simulink library "vmc"  (R2021b)
settings: Solver=VariableStepAuto  StartTime=0.0  StopTime=10.0  RelTol=1e-3
undefined symbols (not defined in the file or in its folder): AVMC_ACCDeltaTqIGain_X_kph, AVMC_ACCDeltaTqIGain_Y_mps2, AVMC_ACCDeltaTqPGain_X_kph, AVMC_ACCDeltaTqPGain_Y_kph, AVMC_ACCLongSteadyCtrl_X_kph, AVMC_AggressJerkPCT4AT_X_kph, AVMC_AggressJerkPCT_X_kph, AVMC_AggressLimitPCT4AT_X_kph, AVMC_AggressLimitPCT_X_kph, AVMC_CCLongSteadyCtrl_X_kph, AVMC_DISCDeltaTqIGain_X_kph, AVMC_DISCDeltaTqIGain_Y_mps2, AVMC_DISCDeltaTqPGain_X_kph, AVMC_DISCDeltaTqPGain_Y_kph, AVMC_DISCTrunAccJerk_X_s, AVMC_DISCTrunAccLimit_X_s, AVMC_ESCRegenOut_X_kph, AVMC_ESCRegenOut_Y_Deg, AVMC_ESCRegenOutEnSpd_X_Deg, AVMC_ISOAccLimit_X_mps, AVMC_ISODecLimit_X_mps, AVMC_ISOJerk_X_mps, AVMC_LatESCRegenOut_X_kph, AVMC_LatESCRegenOut_Y_Deg, AVMC_LongAccDeadZone_X_kph, AVMC_LongAccFiltTsforP2_X_Gps, AVMC_MCPresBaseTq_X_bar, AVMC_MSALongSteadyCtrl_X_kph, AVMC_MSAPedalOvrd2_X_kph, AVMC_MSAPedalOvrd_X_kph, AVMC_MSASpdBand_X_kph, AVMC_MSATqDownEndTq_X_kph, AVMC_MSATqDownTime_X_kph, AVMC_RDCDetectTime_X_kph, AVMC_RDCDetectTime_Y_pct, AVMC_RDCEnSlideRate_X_Deg, AVMC_RearWhlTqRatio_X_Nm, AVMC_RearWhlTqRatio_Y_gps, AVMC_RearWhlTqSlipGain_X_rat, AVMC_RearWhlTqSlipGain_Y_kph, AVMC_SoftJerkPCT_X_kph, AVMC_SoftLimitPCT_X_kph, AVMC_StESCYaw_X_kph, AVMC_StESCYaw_Y_Deg, AVMC_StESCYawCom_X_kph, AVMC_StESCYawCom_Y_Gps, AVMC_TMSpdBaseTq_X_rpm, AVMC_VehHoldBDecMap_X_kph, AVMC_VehHoldDecCtrlTime_X_kph, AVMC_VehHoldMCPPass_X_deg, C_TASK_10MS_S, C_TASK_5MS_S, DEG2RAD, Discrete, ENUM_ACCAVAIL_AVAILABLE, ENUM_ACCCTRLALLOW_ALLOW, ENUM_ADASACCSTA_ACTIVE, ENUM_ADASACCSTA_OVERRIDE, ENUM_ADASACCSTA_SHUTOFF, ENUM_ADASAEBREQ_NOREQUEST ... (+361)
libraries: hcu_lib x63, simulink x60, simulink_extras x3, ctrlSharedLib x3, $bdroot x2
(part 15 of 15)

== stateflow chart vmc/VMC/VMC/SafetyControl/SafetyControlJudgement/SingleWheelSlipRatio/SingleWheelSlipRatioJudgement ==
  state SingleWheelSlipRatioJudgement
    (default) -> (junction 14) : {VVMC_SingleWhlSlipRatioCtrl_flg = FALSE}
    SingleWheelSlipRatioJudgement -> (junction 14)
    (junction 14) -> (junction 105) [order 1] : [VINP_LFRawWhlSpeedV_flg == FALSE]
    (junction 105) -> (junction 117) [order 1] : [abs(VINP_VehSpeed_kph - VVMC_LFWhlSpeedRollAve_kph) >= KVMC_SingleWhlSlipRatioTHR_kph]
    (junction 14) -> (junction 121) [order 2]
    (junction 105) -> (junction 119) [order 2]
    (junction 117) -> (junction 107) : {VVMC_SingleWhlSlipRatioCtrl_flg = TRUE}
    (junction 119) -> (junction 121)
    (junction 121) -> (junction 134)
    (junction 134) -> (junction 130) [order 1] : [VINP_RFRawWhlSpeedV_flg == FALSE]
    (junction 130) -> (junction 125) [order 1] : [abs(VINP_VehSpeed_kph - VVMC_RFWhlSpeedRollAve_kph) >= KVMC_SingleWhlSlipRatioTHR_kph]
    (junction 134) -> (junction 127) [order 2]
    (junction 130) -> (junction 132) [order 2]
    (junction 125) -> (junction 131) : {VVMC_SingleWhlSlipRatioCtrl_flg = TRUE}
    (junction 132) -> (junction 127)
    (junction 127) -> (junction 143)
    (junction 143) -> (junction 149) [order 1] : [VINP_LRRawWhlSpeedV_flg == FALSE]
    (junction 149) -> (junction 144) [order 1] : [abs(VINP_VehSpeed_kph - VVMC_LRWhlSpeedRollAve_kph) >= KVMC_SingleWhlSlipRatioTHR_kph]
    (junction 143) -> (junction 137) [order 2]
    (junction 149) -> (junction 146) [order 2]
    (junction 144) -> (junction 148) : {VVMC_SingleWhlSlipRatioCtrl_flg = TRUE}
    (junction 146) -> (junction 137)
    (junction 137) -> (junction 154)
    (junction 154) -> (junction 153) [order 1] : [VINP_RRRawWhlSpeedV_flg == FALSE]
    (junction 153) -> (junction 150) [order 1] : [abs(VINP_VehSpeed_kph - VVMC_RRWhlSpeedRollAve_kph) >= KVMC_SingleWhlSlipRatioTHR_kph]
    (junction 154) -> (junction 169) [order 2]
    (junction 153) -> (junction 152) [order 2]
    (junction 150) -> (junction 155) : {VVMC_SingleWhlSlipRatioCtrl_flg = TRUE}
    (junction 152) -> (junction 169)
    (junction 169) -> (junction 157)
    (junction 157) -> (junction 163) [order 1] : [(VINP_LFRawWhlSpeedV_flg == TRUE &&...
        |   VINP_RFRawWhlSpeedV_flg == TRUE) ||...
        |  (VINP_LRRawWhlSpeedV_flg == TRUE &&...
        |   VINP_RRRawWhlSpeedV_flg == TRUE)]
    (junction 157) -> (junction 167) [order 2] : {VVMC_SingleWhlSlipRatioCtrl_flg = FALSE}
    (junction 163) -> (junction 165) : {VVMC_SingleWhlSlipRatioCtrl_flg = TRUE}
  data: VINP_VehSpeed_kph input single; VVMC_LFWhlSpeedRollAve_kph input single; VVMC_RFWhlSpeedRollAve_kph input single; VVMC_LRWhlSpeedRollAve_kph input single; VVMC_RRWhlSpeedRollAve_kph input single; VINP_LFRawWhlSpeedV_flg input boolean; VINP_RFRawWhlSpeedV_flg input boolean; VINP_LRRawWhlSpeedV_flg input boolean; VINP_RRRawWhlSpeedV_flg input boolean; KVMC_SingleWhlSlipRatioTHR_kph input single; TRUE input boolean; VVMC_SingleWhlSlipRatioCtrl_flg output boolean; FALSE input boolean

== stateflow chart vmc/VMC/VMC/SpeedArbitration/Response Gain/Response Gain ==
  state ResponseGain
    (default) -> (junction 81) : {VVMC_JerkPCT_pct = ZERO_FLOAT;
        |  VVMC_LimitPCT_pct = ZERO_FLOAT}
    ResponseGain -> (junction 81)
    (junction 81) -> (junction 73) [order 1] : [VVMC_FeatArbitrSta_enum == ENUM_FEATARBITRSTA_DISC ||...
        |  VVMC_FeatArbitrSta_enum == ENUM_FEATARBITRSTA_CC ||...
        |  VVMC_FeatArbitrSta_enum == ENUM_FEATARBITRSTA_MSA ||...
        |  VVMC_FeatArbitrSta_enum == ENUM_FEATARBITRSTA_ACCDISC]
    (junction 73) -> (junction 75) [order 1] : [VDSC_DISCTurn_flg == ENUM_DISCTURN_ACTIVE ||...
        | (VVMC_FeatArbitrSta_enum == ENUM_FEATARBITRSTA_MSA &&...
        |  KVMC_MSAResponseAGSV_flg == TRUE)]
    (junction 81) -> (junction 92) [order 2] : {VVMC_JerkPCT_pct = ZERO_FLOAT;
        |  VVMC_LimitPCT_pct = ZERO_FLOAT}
    (junction 73) -> (junction 77) [order 2] : {VVMC_JerkPCT_pct = VVMC_SoftJerkPCT_pct;
        |  VVMC_LimitPCT_pct = VVMC_SoftLimitPCT_pct}
    (junction 75) -> (junction 78) : {VVMC_JerkPCT_pct = VVMC_AggressJerkPCT_pct;
        |  VVMC_LimitPCT_pct = VVMC_AggressLimitPCT_pct}
  data: VDSC_DISCTurn_flg input uint8; VVMC_FeatArbitrSta_enum input uint8; VVMC_JerkPCT_pct output single; VVMC_LimitPCT_pct output single; VVMC_SoftJerkPCT_pct input single; VVMC_AggressJerkPCT_pct input single; VVMC_SoftLimitPCT_pct input single; VVMC_AggressLimitPCT_pct input single; ENUM_FEATARBITRSTA_DISC input uint8; ENUM_FEATARBITRSTA_CC input; ZERO_FLOAT input single; ENUM_DISCTURN_ACTIVE input uint8; ENUM_FEATARBITRSTA_ACCDISC input uint8; ENUM_FEATARBITRSTA_MSA input; TRUE input; KVMC_MSAResponseAGSV_flg input

== stateflow chart vmc/VMC/VMC/SpeedArbitration/Feature Status Confirm/Feature Status Confirm ==
  state FeatStaConfrim
    (default) -> (junction 197) : {VVMC_FeatStaConfirm_enum = ENUM_FEATSTACFM_INACTIVE}
    FeatStaConfrim -> (junction 197)
    (junction 197) -> (junction 203) [order 1] : [VVMC_VMCAEBCtrlAvail_flg == ENUM_VMCAEBCTRLAVAIL_AVAILABLE &&...
        | (VINP_ADASAEBSta_enum == ENUM_ADASAEBSTA_ACTIVE ||...
        |  VINP_ADASAEBReq_enum ~= ENUM_ADASAEBREQ_NOREQUEST)]
    (junction 197) -> (junction 200) [order 2]
    (junction 203) -> (junction 202) : {VVMC_FeatStaConfirm_enum = ENUM_FEATSTACFM_AEB}
    (junction 200) -> (junction 208) [order 1] : [VVMC_VMCACCCtrlAvail_flg == ENUM_VMCACCCTRLAVAIL_AVAILABLE &&...
        |  VDSC_DISCSta_enum == ENUM_DISCSTA_ACTIVE]
    (junction 208) -> (junction 210) [order 1] : [VINP_ADASACCSta_enum == ENUM_ADASACCSTA_ACTIVE ||...
        |  VINP_ADASACCSta_enum == ENUM_ADASACCSTA_SHUTOFF ||...
        |  VINP_ADASACCSta_enum == ENUM_ADASACCSTA_OVERRIDE]
    (junction 200) -> (junction 232) [order 2]
    (junction 208) -> (junction 214) [order 2]
    (junction 210) -> (junction 212) : {VVMC_FeatStaConfirm_enum = ENUM_FEATSTACFM_ACCDISC}
    (junction 214) -> (junction 216) [order 1] : [(VVMC_CCCtrlSta_enum == ENUM_CCCRLSTA_ACTIVE ||...
        |   VVMC_CCCtrlSta_enum == ENUM_CCCRLSTA_OVERRIDE) &&...
        |  VVMC_VMCCCCtrlAvail_flg == ENUM_VMCCCCTRLAVAIL_AVAILABLE]
    (junction 214) -> (junction 222) [order 2]
    (junction 216) -> (junction 218) : {VVMC_FeatStaConfirm_enum = ENUM_FEATSTACFM_CCDISC}
    (junction 222) -> (junction 224) [order 1] : [(VVMC_MSACtrlSta_enum == ENUM_MSACRLSTA_ACTIVE ||...
        |   VVMC_MSACtrlSta_enum == ENUM_MSACRLSTA_OVERRIDE) &&...
        |  VVMC_VMCMSACtrlAvail_flg == ENUM_VMCMSACTRLAVAIL_AVAILABLE]
    (junction 222) -> (junction 229) [order 2] : {VVMC_FeatStaConfirm_enum = ENUM_FEATSTACFM_DISC}
    (junction 224) -> (junction 221) : {VVMC_FeatStaConfirm_enum = ENUM_FEATSTACFM_DISCMSA}
    (junction 232) -> (junction 234) [order 1] : [VVMC_VMCACCCtrlAvail_flg == ENUM_VMCACCCTRLAVAIL_AVAILABLE &&...
        | (VINP_ADASACCSta_enum == ENUM_ADASACCSTA_ACTIVE ||...
        |  VINP_ADASACCSta_enum == ENUM_ADASACCSTA_OVERRIDE ||...
        |  VINP_ADASACCSta_enum == ENUM_ADASACCSTA_SHUTOFF)]
    (junction 232) -> (junction 238) [order 2]
    (junction 234) -> (junction 236) : {VVMC_FeatStaConfirm_enum = ENUM_FEATSTACFM_ACC}
    (junction 238) -> (junction 240) [order 1] : [(VVMC_CCCtrlSta_enum == ENUM_CCCRLSTA_ACTIVE ||...
        |   VVMC_CCCtrlSta_enum == ENUM_CCCRLSTA_OVERRIDE) &&...
        |  VVMC_VMCCCCtrlAvail_flg == ENUM_VMCCCCTRLAVAIL_AVAILABLE]
    (junction 238) -> (junction 250) [order 2]
    (junction 240) -> (junction 244) : {VVMC_FeatStaConfirm_enum = ENUM_FEATSTACFM_CC}
    (junction 250) -> (junction 249) [order 1] : [(VVMC_MSACtrlSta_enum == ENUM_MSACRLSTA_ACTIVE ||...
        |   VVMC_MSACtrlSta_enum == ENUM_MSACRLSTA_OVERRIDE) &&...
        |  VVMC_VMCMSACtrlAvail_flg == ENUM_VMCMSACTRLAVAIL_AVAILABLE]
    (junction 250) -> (junction 252) [order 2] : {VVMC_FeatStaConfirm_enum = ENUM_FEATSTACFM_INACTIVE}
    (junction 249) -> (junction 248) : {VVMC_FeatStaConfirm_enum = ENUM_FEATSTACFM_MSA}
  data: VVMC_VMCCCCtrlAvail_flg input boolean; ENUM_VMCCCCTRLAVAIL_AVAILABLE input uint8; VVMC_VMCMSACtrlAvail_flg input boolean; ENUM_VMCMSACTRLAVAIL_AVAILABLE input uint8; VVMC_VMCAEBCtrlAvail_flg input boolean; ENUM_VMCAEBCTRLAVAIL_AVAILABLE input uint8; VVMC_VMCACCCtrlAvail_flg input boolean; ENUM_VMCACCCTRLAVAIL_AVAILABLE input uint8; VINP_ADASAEBSta_enum input uint8; VDSC_DISCSta_enum input uint8; VINP_ADASACCSta_enum input uint8; VVMC_CCCtrlSta_enum input uint8; VVMC_FeatStaConfirm_enum output uint8; VVMC_MSACtrlSta_enum input uint8; ENUM_FEATSTACFM_INACTIVE input uint8; ENUM_FEATSTACFM_AEB input uint8; ENUM_FEATSTACFM_ACC input uint8; ENUM_FEATSTACFM_CC input uint8; ENUM_FEATSTACFM_DISC input uint8; ENUM_FEATSTACFM_MSA input uint8; ENUM_FEATSTACFM_ACCDISC input uint8; ENUM_FEATSTACFM_CCDISC input uint8; ENUM_FEATSTACFM_DISCMSA input uint8; ENUM_ADASAEBSTA_ACTIVE input uint8; ENUM_ADASACCSTA_ACTIVE input uint8; ENUM_ADASACCSTA_SHUTOFF input uint8; ENUM_CCCRLSTA_ACTIVE input uint8; ENUM_MSACRLSTA_ACTIVE input uint8; ENUM_DISCSTA_ACTIVE input uint8; ENUM_ADASACCSTA_OVERRIDE input uint8; VINP_ADASAEBReq_enum input uint8; ENUM_ADASAEBREQ_NOREQUEST input uint8; ENUM_CCCRLSTA_OVERRIDE input; ENUM_MSACRLSTA_OVERRIDE input

== stateflow chart vmc/VMC/VMC/SpeedArbitration/Feature Arbitration/Feature Arbitration ==
  state FeatureArbitration
    (default) -> (junction 406) : {VVMC_FeatArbitrSta_enum = ENUM_FEATARBITRSTA_INACTIVE;
        |  VVMC_FeatReqSpd_kph = ZERO_FLOAT;}
    FeatureArbitration -> (junction 406)
    (junction 406) -> (junction 409) [order 1] : [VVMC_FeatStaConfirm_enum == ENUM_FEATSTACFM_AEB]
    (junction 406) -> (junction 413) [order 2]
    (junction 409) -> (junction 411) : {VVMC_FeatArbitrSta_enum = ENUM_FEATARBITRSTA_AEB;
        |  VVMC_FeatReqSpd_kph = ZERO_FLOAT}
    (junction 413) -> (junction 415) [order 1] : [VVMC_FeatStaConfirm_enum == ENUM_FEATSTACFM_ACC]
    (junction 413) -> (junction 430) [order 2]
    (junction 415) -> (junction 417) : {VVMC_FeatArbitrSta_enum = ENUM_FEATARBITRSTA_ACC;
        |  VVMC_FeatReqSpd_kph = ZERO_FLOAT}
    (junction 430) -> (junction 431) [order 1] : [VVMC_FeatStaConfirm_enum == ENUM_FEATSTACFM_CC]
    (junction 430) -> (junction 440) [order 2]
    (junction 431) -> (junction 433) : {VVMC_FeatArbitrSta_enum = ENUM_FEATARBITRSTA_CC;
        |  VVMC_FeatReqSpd_kph = VVMC_FeatSetSpdForCalcu_kph}
    (junction 440) -> (junction 441) [order 1] : [VVMC_FeatStaConfirm_enum == ENUM_FEATSTACFM_DISC]
    (junction 440) -> (junction 445) [order 2]
    (junction 441) -> (junction 438) : {VVMC_FeatArbitrSta_enum = ENUM_FEATARBITRSTA_DISC;
        |  VVMC_FeatReqSpd_kph = VDSC_DISCTargetSpd_kph}
    (junction 445) -> (junction 443) [order 1] : [VVMC_FeatStaConfirm_enum == ENUM_FEATSTACFM_MSA]
    (junction 445) -> (junction 449) [order 2]
    (junction 443) -> (junction 444) : {VVMC_FeatArbitrSta_enum = ENUM_FEATARBITRSTA_MSA;
        |  VVMC_FeatReqSpd_kph = VVMC_FeatSetSpdForCalcu_kph}
    (junction 449) -> (junction 450) [order 1] : [VVMC_FeatStaConfirm_enum == ENUM_FEATSTACFM_ACCDISC]
    (junction 450) -> (junction 557) [order 1] : [VVMC_FeatSetSpdForCalcu_kph <= VDSC_DISCTargetSpd_kph]
    (junction 557) -> (junction 551) [order 1] : [VVMC_FeatSetSpdForCalcu_kph < VDSC_DISCTargetSpd_kph]
    (junction 449) -> (junction 512) [order 2]
    (junction 450) -> (junction 467) [order 2] : {VVMC_FeatArbitrSta_enum = ENUM_FEATARBITRSTA_ACCDISC;
        |  VVMC_FeatReqSpd_kph = VDSC_DISCTargetSpd_kph}
    (junction 557) -> (junction 559) [order 2]
    (junction 551) -> (junction 553) : {VVMC_FeatArbitrSta_enum = ENUM_FEATARBITRSTA_ACC;
        |  VVMC_FeatReqSpd_kph = ZERO_FLOAT}
    (junction 559) -> (junction 561) [order 1] : [VVMC_LastFeatArbitrFinal_enum != ENUM_FEATARBITRSTA_DISC]
    (junction 559) -> (junction 565) [order 2]
    (junction 561) -> (junction 564) : {VVMC_FeatArbitrSta_enum = ENUM_FEATARBITRSTA_ACC;
        |  VVMC_FeatReqSpd_kph = ZERO_FLOAT}
    (junction 565) -> (junction 567) [order 1] : [VVMC_LastActACCRequiredAccel_mps2 > ZERO_FLOAT ||...
        |  VVMC_LastActACCRequiredAccel_mps2 < ZERO_FLOAT ]
    (junction 565) -> (junction 569) [order 2] : {VVMC_FeatArbitrSta_enum = ENUM_FEATARBITRSTA_ACC;
        |  VVMC_FeatReqSpd_kph = ZERO_FLOAT}
    (junction 567) -> (junction 572) : {VVMC_FeatArbitrSta_enum = ENUM_FEATARBITRSTA_DISC;
        |  VVMC_FeatReqSpd_kph = VDSC_DISCTargetSpd_kph}
    (junction 512) -> (junction 514) [order 1] : [VVMC_FeatStaConfirm_enum == ENUM_FEATSTACFM_CCDISC ||...
        |  VVMC_FeatStaConfirm_enum == ENUM_FEATSTACFM_DISCMSA]
    (junction 514) -> (junction 516) [order 1] : [VVMC_FeatSetSpdForCalcu_kph < VDSC_DISCTargetSpd_kph]
    (junction 516) -> (junction 518) [order 1] : [VVMC_FeatStaConfirm_enum == ENUM_FEATSTACFM_CCDISC]
    (junction 512) -> (junction 527) [order 2] : {VVMC_FeatArbitrSta_enum = ENUM_FEATARBITRSTA_INACTIVE;
        |  VVMC_FeatReqSpd_kph = ZERO_FLOAT}
    (junction 514) -> (junction 525) [order 2] : {VVMC_FeatArbitrSta_enum = ENUM_FEATARBITRSTA_DISC;
        |  VVMC_FeatReqSpd_kph = VDSC_DISCTargetSpd_kph}
    (junction 516) -> (junction 522) [order 2] : {VVMC_FeatArbitrSta_enum = ENUM_FEATARBITRSTA_MSA;
        |  VVMC_FeatReqSpd_kph = VVMC_FeatSetSpdForCalcu_kph}
    (junction 518) -> (junction 520) : {VVMC_FeatArbitrSta_enum = ENUM_FEATARBITRSTA_CC;
        |  VVMC_FeatReqSpd_kph = VVMC_FeatSetSpdForCalcu_kph}
  data: VVMC_FeatStaConfirm_enum input uint8; VDSC_DISCTargetSpd_kph input single; VVMC_FeatSetSpdForCalcu_kph input single; VVMC_FeatArbitrSta_enum output uint8; VVMC_FeatReqSpd_kph output single; ENUM_FEATSTACFM_AEB input uint8; ENUM_FEATSTACFM_ACC input uint8; ENUM_FEATSTACFM_CC input uint8; ENUM_FEATSTACFM_DISC input uint8; ENUM_FEATSTACFM_MSA input uint8; ENUM_FEATSTACFM_ACCDISC input uint8; ENUM_FEATSTACFM_CCDISC input uint8; ENUM_FEATSTACFM_DISCMSA input uint8; ENUM_FEATARBITRSTA_INACTIVE input uint8; ENUM_FEATARBITRSTA_AEB input uint8; ENUM_FEATARBITRSTA_ACC input uint8; ENUM_FEATARBITRSTA_CC input uint8; ENUM_FEATARBITRSTA_DISC input uint8; ENUM_FEATARBITRSTA_ACCDISC input uint8; ENUM_FEATARBITRSTA_MSA input uint8; ZERO_FLOAT input single; VVMC_LastActACCRequiredAccel_mps2 input; VVMC_LastFeatArbitrFinal_enum input
